simulink model "Problem7"  (R2020a)
settings: Solver=VariableStepAuto  StartTime=0.0  StopTime=10.0  RelTol=1e-3
model workspace (MAT data in the model file):
  A = Simulink.Parameter
  A.Value = 2
  A.DataType = 'auto'
  A.Dimensions = [1 1]
  B = Simulink.Parameter
  B.Value = -3
  B.DataType = 'auto'
  B.Dimensions = [1 1]
  C = Simulink.Parameter
  C.Value = -4
  C.DataType = 'auto'
  C.Dimensions = [1 1]
  D = Simulink.Parameter
  D.Value = 5
  D.DataType = 'auto'
  D.Dimensions = [1 1]
libraries: dspsrcs4 x1
settings Model: Creator=Admin  LastModifiedBy=Admin

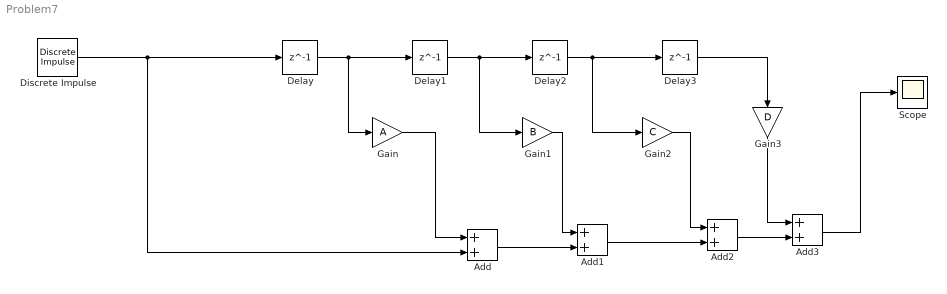
== system Problem7 ==
  Add{,1..3} (4 alike) : Sum
  Delay{,1..3} (4 alike) : Delay  DelayLength=1
  Discrete Impulse : dspsrcs4/Discrete  Impulse  Delay=0  SampleTime=1  FrameSample=1  OutputFrames=off  dataType=double  isSigned=on  wordLen=16  udDataType=sfix(16)  fracBitsMode=Best precision  numFracBits=15  OutDataTypeStr=double  LastOutDataTypeStr=double
  Gain : Gain  Gain=A
  Gain1 : Gain  Gain=B
  Gain2 : Gain  Gain=C
  Gain3 : Gain  Gain=D
  Scope : Scope
  wires:
  Discrete Impulse/1 -> Add/2, Delay/1
  Delay/1 -> Gain/1, Delay1/1
  Gain/1 -> Add/1
  Delay1/1 -> Gain1/1, Delay2/1
  Delay2/1 -> Gain2/1, Delay3/1
  Add/1 -> Add1/2
  Gain1/1 -> Add1/1
  Add1/1 -> Add2/2
  Gain2/1 -> Add2/1
  Delay3/1 -> Gain3/1
  Add2/1 -> Add3/2
  Gain3/1 -> Add3/1
  Add3/1 -> Scope/1
